simulink model "CiaglyUkladstary"  (Simulink 10.1)
settings: Solver=VariableStepAuto  StartTime=0.0  StopTime=1  MaxStep=1e-3  MinStep=1e-4  RelTol=1e-3
values from neighbouring files (symbols this model uses):
  In = 141    [Parametry.m]
  J = Js    (= 0.97)    [Parametry.m]
  Kp = 1.5*Un / 10    (= 34.5)    [Parametry.m]
  Kri = T*Rt / (2*Kp*Y*tau0)    (= 0.252338603426)    [Parametry.m]
  Krw = J*Y / (4*Kt*tau0*psien)    (= 7.34565732899)    [Parametry.m]
  Kt = 10 / (1.2*wn)    (= 0.109762029719)    [Parametry.m]
  lambdan = 2    [Parametry.m]
  Mn = In * psien    (= 364.565023633)    [Parametry.m]
  psien = (Un-In*Rt)/wn    (= 2.58556754349)    [Parametry.m]
  Rt = 0.239    [Parametry.m]
  T = Lt/Rt    (= 0.00682008368201)    [Parametry.m]
  Tri = T    (= 0.00682008368201)    [Parametry.m]
  Trw = 8*tau0    (= 0.0264)    [Parametry.m]
  uz0 = lambdan*In/kz    (= 8)    [Parametry.m]
  wn = nn*2*pi/60    (= 75.9218224618)    [Parametry.m]
  Y = 10 / (2.5*In)    (= 0.0283687943262)    [Parametry.m]
settings Model: Creator=Admin  LastModifiedBy=Admin
settings SolverCC: InitialStep=1e-4
settings DataIOCC: SaveFormat=Dataset  ReturnWorkspaceOutputs=on
settings OptimizationCC: LifeSpan=auto
settings DebuggingCC: UnderspecifiedInitializationDetection=Simplified  MergeDetectMultiDrivingBlocksExec=error  SFUnexpectedBacktrackingDiag=error  SFNoUnconditionalDefaultTransitionDiag=error  SFExecutionAtInitializationDiag=warning
settings HardwareCC: ProdBitPerPointer=64  ProdBitPerSizeT=64  ProdBitPerPtrDiffT=64  ProdLargestAtomicFloat=Float  ProdIntDivRoundTo=Zero  ProdEndianess=LittleEndian  ProdWordSize=64  ProdHWDeviceType=Intel->x86-64 (Windows64)
settings ModelReferenceCC: PropagateSignalLabelsOutOfModel=on
settings SFSimCC: SimUseLocalCustomCode=on
settings RTWCC: RTWUseLocalCustomCode=on
settings CodeAppCC: StateflowObjectComments=off
settings GRTTargetCC: TargetLangStandard=C99 (ISO)  CombineOutputUpdateFcns=on  GRTInterface=off
settings ConfigComp: CovMetricSettings=dwe  CovHtmlReporting=off  CovSaveCumulativeToWorkspaceVar=off  CovSaveSingleToWorkspaceVar=off  CovExternalEMLEnable=on

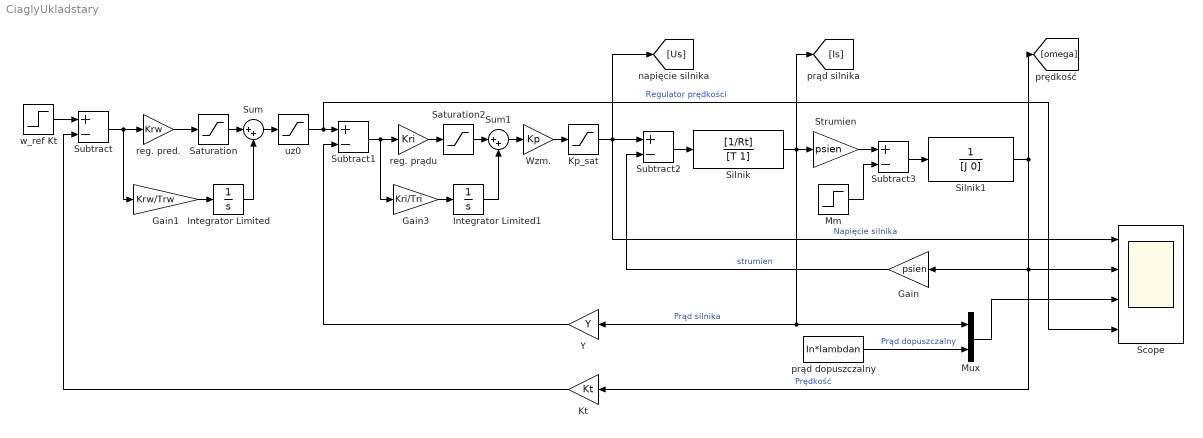
== system CiaglyUkladstary ==
  Gain : Gain  Gain=psien
  Gain1 : Gain  Gain=Krw/Trw
  Gain3 : Gain  Gain=Kri/Tri
  Integrator Limited : Integrator  LimitOutput=on  UpperSaturationLimit=10  LowerSaturationLimit=-10
  Integrator Limited1 : Integrator  LimitOutput=on  UpperSaturationLimit=10  LowerSaturationLimit=-10
  Kp_sat : Saturate  UpperLimit=700  LowerLimit=-700
  Kt : Gain  Gain=Kt
  Mm : Step  Time=0  After=Mn  SampleTime=0
  Mux : Mux  Inputs=2
  Saturation : Saturate  UpperLimit=10  LowerLimit=-10
  Saturation2 : Saturate  UpperLimit=10  LowerLimit=-10
  Scope : Scope  NumInputPorts=4
  Silnik : TransferFcn  Numerator=[1/Rt]  Denominator=[T 1]
  Silnik1 : TransferFcn  Denominator=[J 0]
  Strumien : Gain  Gain=psien
  Subtract{,1..3} (4 alike) : Sum  Inputs=+-
  Sum : Sum  Inputs=|++
  Sum1 : Sum  Inputs=|++
  Wzm. : Gain  Gain=Kp
  Y : Gain  Gain=Y
  prąd dopuszczalny : Constant  Value=In*lambdan
  reg. pred. : Gain  Gain=Krw
  reg. prądu : Gain  Gain=Kri
  uz0 : Saturate  UpperLimit=uz0  LowerLimit=-uz0
  w_ref Kt : Step  Time=0  After=wn  SampleTime=0
  wires:
  Subtract/1 -> Gain1/1, reg. pred./1
  Gain1/1 -> Integrator Limited/1
  Integrator Limited/1 -> Sum/2
  Saturation/1 -> Sum/1
  reg. pred./1 -> Saturation/1
  Sum/1 -> uz0/1
  reg. prądu/1 -> Saturation2/1
  Subtract1/1 -> reg. prądu/1, Gain3/1
  Saturation2/1 -> Sum1/1
  Gain3/1 -> Integrator Limited1/1
  Integrator Limited1/1 -> Sum1/2
  Sum1/1 -> Wzm./1
  Wzm./1 -> Kp_sat/1
  Subtract2/1 -> Silnik/1
  w_ref Kt/1 -> Subtract/1
  Silnik/1 -> Y/1, Mux/1, [Is], Strumien/1  "Prąd silnika"
  Strumien/1 -> Subtract3/1
  Mm/1 -> Subtract3/2
  Subtract3/1 -> Silnik1/1
  Gain/1 -> Subtract2/2  "strumien"
  Y/1 -> Subtract1/2
  Kt/1 -> Subtract/2
  Kp_sat/1 -> Subtract2/1, [Us], Scope/1  "Napięcie silnika"
  Silnik1/1 -> Scope/2, Gain/1, Kt/1, [omega]  "Prędkość"
  uz0/1 -> Scope/4, Subtract1/1  "Regulator prędkości"
  prąd dopuszczalny/1 -> Mux/2  "Prąd dopuszczalny"
  Mux/1 -> Scope/3
